simulink model "ex_model1_fixed"  (R2022b)
settings: configuration reference "Configuration" (kept outside this file)
libraries: FixedLib x2
settings Model: Creator=amyyang  LastModifiedBy=amyyang
settings ConfigSetRef: SourceName=Configuration  SourceLocation=Base Workspace

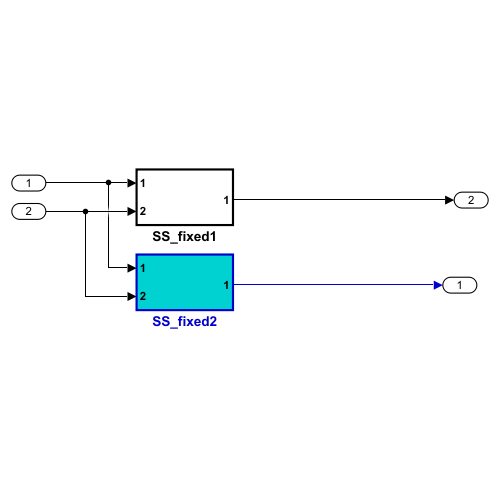
[thumbnail: Simulink's stored preview of the top-level diagram]
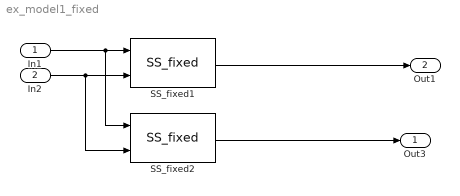
== system ex_model1_fixed ==
  In1 : Inport
  In2 : Inport  Port=2
  SS_fixed1 : FixedLib/SS_fixed  x=T1Break  y=T1Data
  SS_fixed2 : FixedLib/SS_fixed  x=T1Break  y=T1Data
  Out3 : Outport
  Out1 : Outport  Port=2
  wires:
  In1/1 -> SS_fixed1/1, SS_fixed2/1
  In2/1 -> SS_fixed2/2, SS_fixed1/2
  SS_fixed1/1 -> Out1/1
  SS_fixed2/1 -> Out3/1
